simulink model "gm_sampleModel1847_2_sub_sub_sub"  (R2023a)
settings: Solver=VariableStepAuto  StartTime=0.0  StopTime=10.0  RelTol=1e-3
libraries: hdlsllib x3
settings Model: Creator=user1  LastModifiedBy=user1
settings OptimizationCC: BlockReduction=off  ConditionallyExecuteInputs=off
settings DebuggingCC: InheritedTsInSrcMsg=none

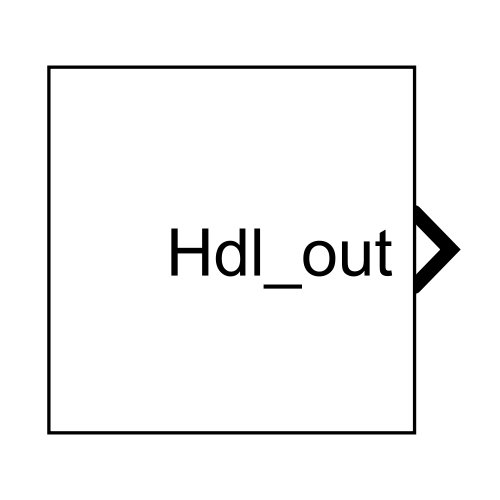
[thumbnail: Simulink's stored preview of the top-level diagram]
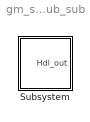
== system gm_sampleModel1847_2_sub_sub_sub ==
  Subsystem : Subsystem

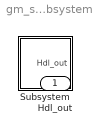
== system gm_sampleModel1847_2_sub_sub_sub/Subsystem ==
  Subsystem : Subsystem
  Hdl_out : Outport  OutDataTypeStr=uint8

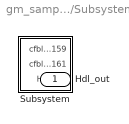
== system gm_sampleModel1847_2_sub_sub_sub/Subsystem/Subsystem ==
  Subsystem : Subsystem
  Hdl_out : Outport  OutDataTypeStr=uint8

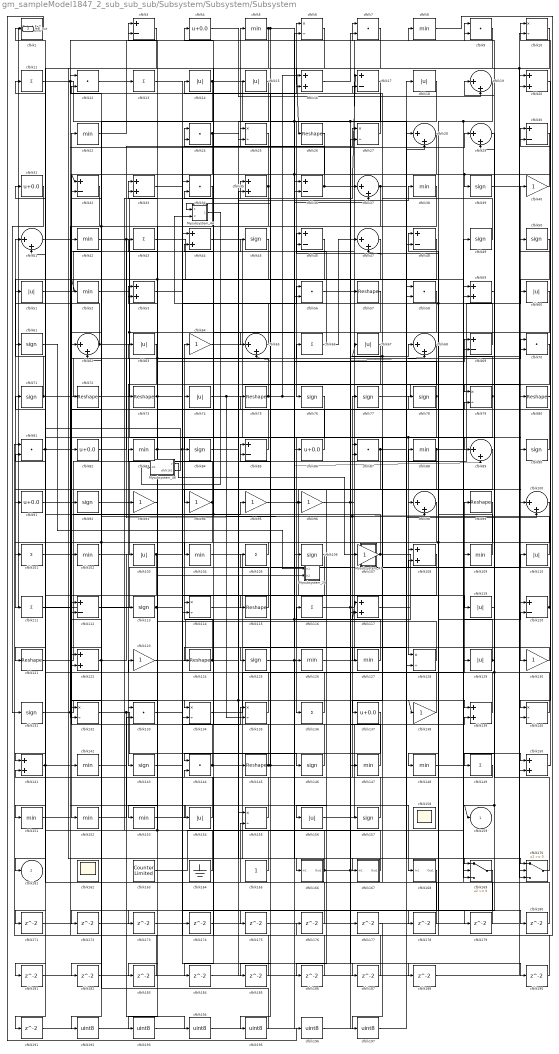
== system gm_sampleModel1847_2_sub_sub_sub/Subsystem/Subsystem/Subsystem ==
  Mysubsystem_26 : Subsystem  TreatAsAtomicUnit=on  RTWFcnName=Mysubsystem_26
      settings: RTWFcnNameOpts=User specified  RTWFileNameOpts=Use function name
  Mysubsystem_43 : Subsystem  TreatAsAtomicUnit=on  RTWFcnName=Mysubsystem_43
      settings: RTWFcnNameOpts=User specified  RTWFileNameOpts=Use function name
  Mysubsystem_44 : Subsystem  TreatAsAtomicUnit=on  RTWFcnName=Mysubsystem_44
      settings: RTWFcnNameOpts=User specified  RTWFileNameOpts=Use function name
  Mysubsystem_46 : Subsystem  TreatAsAtomicUnit=on  RTWFcnName=Mysubsystem_46
      settings: RTWFcnNameOpts=User specified  RTWFileNameOpts=Use function name
  cfblk1 : hdlsllib/Logic and Bit Operations/Detect Fall Nonpositive  vinit=0  OutDataTypeStr=uint8
  cfblk{6,10,25,27,79,114,128,132,134..135,140,155} (12 alike) : Product  Inputs=*/  OutDataTypeStr=uint8  RndMeth=Zero  SaturateOnIntegerOverflow=on
  cfblk{19,28..29,37,41,47,62,65,68,89,98,100} (12 alike) : Sum  Inputs=|++  OutDataTypeStr=uint8
  cfblk{11,13,43,66,101,105,111,116,136,149} (10 alike) : Sum  Inputs=+  OutDataTypeStr=uint8
  cfblk{5,8,22,38,42,52,83,88,102,104,109,126..127,142,147..148,151..153} (19 alike) : MinMax  OutDataTypeStr=uint8
  cfblk{14..15,18,51,60,63,67,74,103,110,119,129,154,156} (14 alike) : Abs  OutDataTypeStr=uint8  SaturateOnIntegerOverflow=off
  cfblk{39,45,49..50,61,71,76..78,84,90,92,106,113,125,131,143,146,157} (19 alike) : Signum
  cfblk{40,64,93..96,107,123,130,138} (10 alike) : Gain  OutDataTypeStr=uint8
  cfblk{16,20,33,35,44,53,59,108,117,122,139,141,150} (13 alike) : Sum  OutDataTypeStr=uint8
  cfblk{3,17,30,32,36,46,48,69,85,112,120} (11 alike) : Sum  Inputs=+-  OutDataTypeStr=uint8
  cfblk{26,57,72..73,75,80,99,115,121,124,145} (11 alike) : Reshape
  cfblk{7,9,12,24,34,56,58,70,81,87,133,144} (12 alike) : DotProduct  OutDataTypeStr=uint8
  cfblk{4,31,82,86,91,137} (6 alike) : Bias  Bias=0.0  SaturateOnIntegerOverflow=off
  cfblk158 : Scope
      settings: Floating=on
  cfblk162 : Scope
      settings: Floating=on
  cfblk163 : hdlsllib/Sources/Counter Limited  uplimit=7  tsamp=-1
  cfblk164 : Ground
  cfblk165 : Constant  OutDataTypeStr=uint8  SampleTime=-1
  cfblk166 : Subsystem
      settings: LibrarySourceBlock=|
      | hdlsllib/Ports &
      | Subsystems/Subsystem
  cfblk167 : Subsystem
      settings: LibrarySourceBlock=|
      | hdlsllib/Ports &
      | Subsystems/Subsystem
  cfblk168 : Subsystem
      settings: LibrarySourceBlock=|
      | hdlsllib/Ports &
      | Subsystems/Subsystem
  cfblk169 : Switch  OutDataTypeStr=uint8  SaturateOnIntegerOverflow=off  InputSameDT=off
  cfblk170 : Switch  OutDataTypeStr=uint8  SaturateOnIntegerOverflow=off  InputSameDT=off
  cfblk{171..188,190..191} (20 alike) : Delay  SampleTime=1
  cfblk{192..197} (6 alike) : DataTypeConversion  OutDataTypeStr=uint8  SaturateOnIntegerOverflow=off  RndMeth=Floor
  cfblk159 : Outport  OutDataTypeStr=uint8  VectorParamsAs1DForOutWhenUnconnected=off
  cfblk161 : Outport  Port=2  OutDataTypeStr=uint8  VectorParamsAs1DForOutWhenUnconnected=off
  Hdl_out : Outport  Port=3  OutDataTypeStr=uint8
  wires:
  Mysubsystem_46/2(cfblk161) -> cfblk161/1
  Mysubsystem_46/1(y) -> Mysubsystem_43/1(In1)
  Mysubsystem_44/1(Out1) -> Mysubsystem_46/1(In1)
  cfblk61/1 -> Mysubsystem_26/1(In1)
  cfblk197/1 -> cfblk58/2
  cfblk177/1 -> cfblk197/1
  cfblk196/1 -> cfblk58/1
  cfblk1/1 -> cfblk196/1
  cfblk195/1 -> cfblk42/1
  cfblk58/1 -> cfblk195/1
  cfblk194/1 -> cfblk28/2
  cfblk193/1 -> cfblk28/1
  cfblk192/1 -> cfblk177/1
  cfblk28/1 -> cfblk192/1
  cfblk191/1 -> cfblk56/2
  cfblk190/1 -> cfblk108/2
  cfblk188/1 -> cfblk120/1
  cfblk187/1 -> cfblk44/1
  cfblk33/1 -> cfblk187/1
  cfblk186/1 -> cfblk144/2
  cfblk98/1 -> cfblk186/1
  cfblk185/1 -> cfblk12/1
  cfblk169/1 -> cfblk185/1
  cfblk184/1 -> cfblk35/2
  cfblk9/1 -> cfblk184/1
  cfblk183/1 -> cfblk81/1
  cfblk182/1 -> cfblk10/2
  cfblk181/1 -> cfblk27/2
  cfblk180/1 -> cfblk59/1
  cfblk179/1 -> cfblk17/2
  cfblk178/1 -> cfblk1/1
  cfblk176/1 -> cfblk155/2
  cfblk8/1 -> cfblk176/1
  cfblk175/1 -> cfblk6/2
  cfblk57/1 -> cfblk175/1
  cfblk174/1 -> cfblk20/2
  cfblk133/1 -> cfblk174/1
  cfblk173/1 -> cfblk34/1
  cfblk93/1 -> cfblk173/1
  cfblk172/1 -> cfblk36/1
  cfblk168/1(Out1) -> cfblk172/1
  cfblk171/1 -> cfblk140/2
  cfblk84/1 -> cfblk167/1(In1), cfblk138/1
  cfblk130/1 -> cfblk124/1
  cfblk69/1 -> cfblk44/2
  cfblk63/1 -> cfblk73/1
  cfblk116/1 -> cfblk30/2, cfblk68/2
  cfblk142/1 -> cfblk169/1
  cfblk13/1 -> cfblk59/2
  cfblk127/1 -> cfblk116/1
  cfblk135/1 -> cfblk51/1
  cfblk4/1 -> cfblk19/2
  cfblk53/1 -> cfblk45/1
  cfblk67/1 -> cfblk115/1
  cfblk49/1 -> cfblk14/1
  cfblk150/1 -> cfblk30/1
  cfblk107/1 -> cfblk81/2, cfblk4/1, cfblk110/1
  cfblk14/1 -> cfblk48/2, cfblk147/1, cfblk132/1
  cfblk136/1 -> cfblk112/2
  cfblk51/1 -> cfblk18/1
  cfblk17/1 -> cfblk65/1
  cfblk83/1 -> cfblk27/1, cfblk96/1, cfblk3/2
  cfblk45/1 -> cfblk52/1, cfblk183/1
  cfblk110/1 -> cfblk87/2, cfblk62/2
  cfblk94/1 -> cfblk122/1, cfblk122/2, cfblk53/2
  cfblk15/1 -> cfblk25/2
  cfblk81/1 -> cfblk79/2, cfblk171/1
  cfblk19/1 -> cfblk148/1, cfblk169/2
  cfblk59/1 -> cfblk19/1
  cfblk111/1 -> cfblk69/1
  cfblk77/1 -> cfblk79/1
  cfblk26/1 -> cfblk36/2, cfblk62/1
  cfblk16/1 -> cfblk7/2
  cfblk75/1 -> cfblk128/2, cfblk16/1, Mysubsystem_26/2(In2), cfblk33/2
  cfblk22/1 -> cfblk7/1
  cfblk165/1 -> cfblk43/1, cfblk32/2
  cfblk65/1 -> cfblk34/2
  cfblk11/1 -> cfblk157/1, cfblk86/1, cfblk16/2
  cfblk41/1 -> cfblk29/1
  cfblk117/1 -> cfblk60/1
  cfblk47/1 -> cfblk134/2
  cfblk140/1 -> cfblk85/2, cfblk109/1
  cfblk70/1 -> cfblk125/1
  cfblk115/1 -> cfblk105/1
  cfblk48/1 -> cfblk102/1
  cfblk6/1 -> cfblk84/1
  cfblk109/1 -> Mysubsystem_44/2(In2), cfblk48/1
  cfblk163/1 -> cfblk129/1
  cfblk12/1 -> cfblk13/1
  cfblk156/1 -> cfblk49/1
  cfblk24/1 -> cfblk112/1, cfblk89/1
  cfblk104/1 -> cfblk127/1
  cfblk88/1 -> cfblk156/1, cfblk150/1
  cfblk90/1 -> cfblk33/1
  cfblk39/1 -> cfblk170/3
  cfblk108/1 -> cfblk151/1
  cfblk151/1 -> cfblk154/1
  cfblk128/1 -> cfblk3/1
  cfblk71/1 -> cfblk41/1, cfblk66/1
  cfblk34/1 -> cfblk113/1
  cfblk101/1 -> cfblk95/1
  cfblk66/1 -> cfblk46/1, cfblk47/1
  cfblk129/1 -> cfblk88/1, cfblk29/2
  cfblk31/1 -> cfblk131/1
  cfblk105/1 -> cfblk101/1
  cfblk95/1 -> cfblk119/1, cfblk100/1
  cfblk91/1 -> cfblk63/1
  cfblk37/1 -> cfblk93/1, cfblk100/2
  cfblk40/1 -> cfblk39/1, cfblk32/1
  cfblk120/1 -> cfblk50/1, cfblk75/1
  cfblk144/1 -> cfblk38/1, cfblk12/2
  cfblk113/1 -> cfblk56/1, Hdl_out/1
  cfblk7/1 -> cfblk91/1
  cfblk96/1 -> cfblk40/1, cfblk68/1, cfblk190/1
  cfblk92/1 -> cfblk70/2
  cfblk103/1 -> cfblk180/1, cfblk181/1
  cfblk25/1 -> cfblk24/2
  cfblk164/1 -> cfblk71/1
  cfblk148/1 -> cfblk120/2
  cfblk143/1 -> cfblk135/1
  cfblk72/1 -> cfblk70/1
  cfblk141/1 -> cfblk8/1, cfblk31/1
  cfblk5/1 -> Mysubsystem_44/1(In1), cfblk37/2, cfblk41/2
  cfblk52/1 -> cfblk114/2, cfblk106/1
  cfblk112/1 -> cfblk57/1
  cfblk123/1 -> cfblk20/1
  cfblk147/1 -> cfblk114/1
  cfblk29/1 -> cfblk149/1
  cfblk43/1 -> cfblk145/1
  cfblk86/1 -> cfblk25/1
  cfblk152/1 -> cfblk133/2
  cfblk89/1 -> cfblk98/1
  cfblk139/1 -> cfblk67/1, cfblk47/2
  cfblk79/1 -> cfblk137/1, cfblk46/2
  cfblk149/1 -> cfblk141/2
  cfblk74/1 -> cfblk108/1, cfblk135/2
  cfblk166/1(Out1) -> cfblk139/2, cfblk188/1, cfblk61/1
  cfblk60/1 -> cfblk94/1
  cfblk138/1 -> cfblk92/1
  cfblk121/1 -> cfblk87/1
  cfblk100/1 -> cfblk104/1
  cfblk122/1 -> cfblk103/1, cfblk182/1
  cfblk20/1 -> cfblk140/1
  cfblk62/1 -> cfblk37/1, cfblk11/1
  cfblk125/1 -> cfblk170/2, cfblk69/2
  cfblk106/1 -> cfblk121/1
  cfblk10/1 -> cfblk26/1, cfblk150/2
  cfblk137/1 -> cfblk144/1
  cfblk38/1 -> cfblk153/1
  cfblk82/1 -> cfblk24/1
  cfblk80/1 -> cfblk10/1
  cfblk42/1 -> cfblk155/1, cfblk98/2
  cfblk145/1 -> cfblk89/2, cfblk117/1, cfblk126/1, cfblk65/2, cfblk72/1
  cfblk56/1 -> cfblk107/1
  cfblk154/1 -> cfblk83/1
  cfblk119/1 -> cfblk159/1, cfblk179/1
  cfblk44/1 -> cfblk90/1
  cfblk32/1 -> cfblk142/1
  cfblk114/1 -> cfblk170/1
  cfblk73/1 -> cfblk133/1, cfblk117/2
  cfblk102/1 -> cfblk85/1
  cfblk76/1 -> cfblk136/1
  cfblk155/1 -> cfblk123/1
  cfblk146/1 -> cfblk22/1
  cfblk157/1 -> cfblk77/1
  cfblk124/1 -> cfblk74/1, cfblk78/1
  cfblk27/1 -> cfblk6/1
  cfblk170/1 -> cfblk9/2
  cfblk87/1 -> cfblk141/1, cfblk169/3
  cfblk36/1 -> cfblk17/1, cfblk15/1
  cfblk126/1 -> cfblk9/1
  cfblk35/1 -> cfblk132/2, cfblk82/1, cfblk5/1
  cfblk131/1 -> cfblk134/1, cfblk139/1
  cfblk18/1 -> cfblk76/1
  cfblk153/1 -> cfblk168/1(In1)
  cfblk46/1 -> cfblk111/1
  cfblk99/1 -> cfblk178/1, cfblk193/1
  cfblk132/1 -> cfblk146/1, cfblk194/1
  cfblk167/1(Out1) -> cfblk35/1
  cfblk3/1 -> cfblk166/1(In1)
  cfblk30/1 -> cfblk152/1
  cfblk134/1 -> cfblk99/1
  cfblk78/1 -> cfblk128/1, cfblk191/1, cfblk53/1
  cfblk85/1 -> cfblk64/1
  cfblk64/1 -> cfblk80/1
  cfblk68/1 -> cfblk143/1
  cfblk50/1 -> cfblk130/1

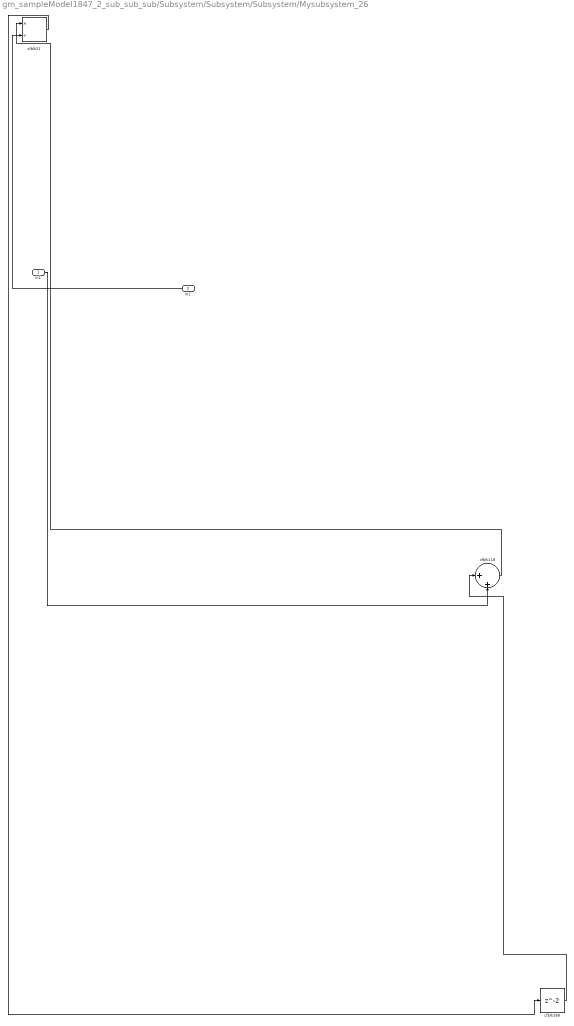
== system gm_sampleModel1847_2_sub_sub_sub/Subsystem/Subsystem/Subsystem/Mysubsystem_26 ==
  In1 : Inport
  In2 : Inport  Port=2
  cfblk118 : Sum  Inputs=|++
  cfblk189 : Delay  SampleTime=1
  cfblk21 : Product  Inputs=*/  RndMeth=Zero  SaturateOnIntegerOverflow=on
  wires:
  cfblk118/1 -> cfblk21/1
  cfblk21/1 -> cfblk189/1
  cfblk189/1 -> cfblk118/1
  In1/1 -> cfblk118/2
  In2/1 -> cfblk21/2

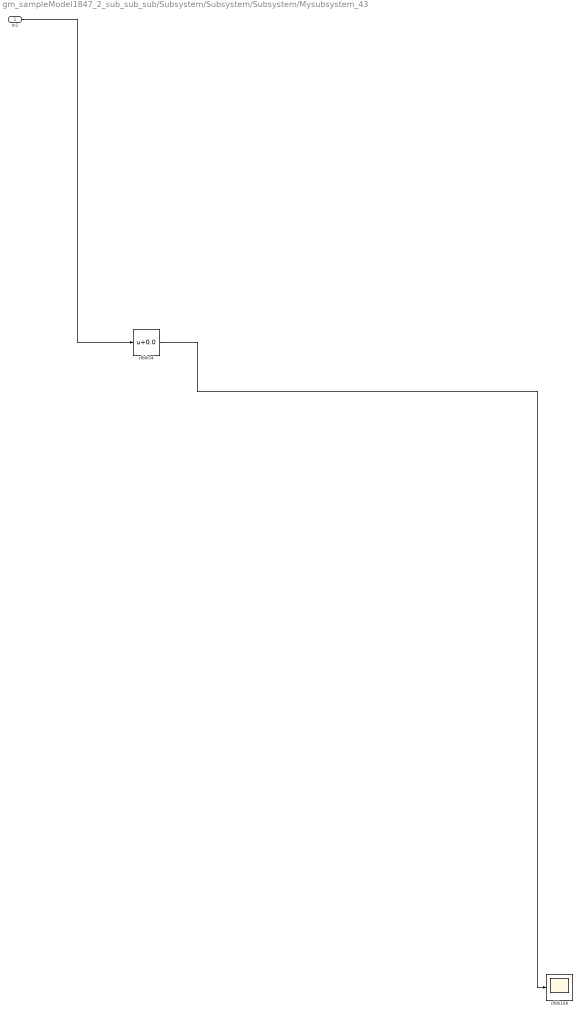
== system gm_sampleModel1847_2_sub_sub_sub/Subsystem/Subsystem/Subsystem/Mysubsystem_43 ==
  In1 : Inport
  cfblk160 : Scope
  cfblk54 : Bias  Bias=0.0  SaturateOnIntegerOverflow=off
  wires:
  cfblk54/1 -> cfblk160/1
  In1/1 -> cfblk54/1

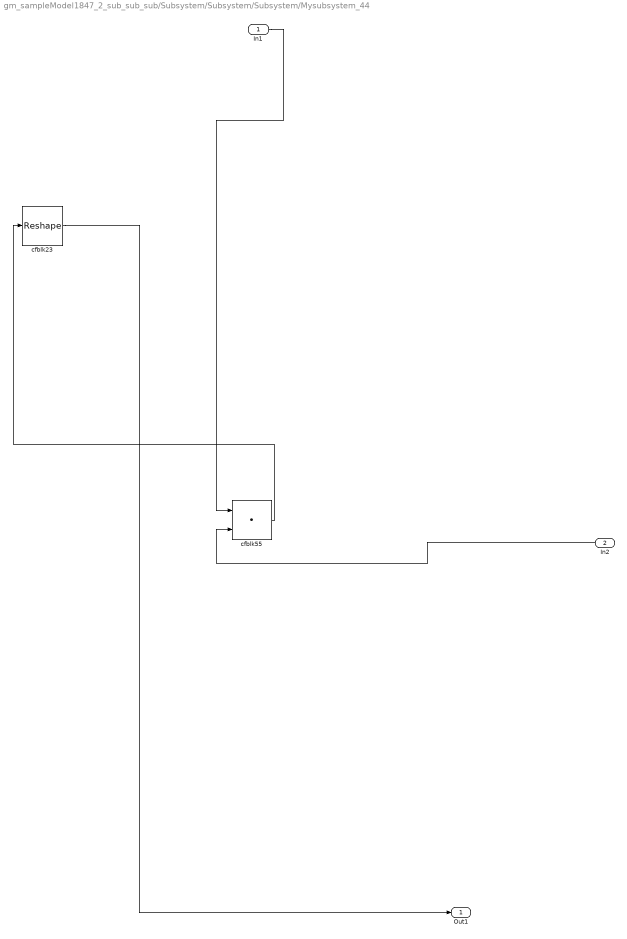
== system gm_sampleModel1847_2_sub_sub_sub/Subsystem/Subsystem/Subsystem/Mysubsystem_44 ==
  In1 : Inport
  In2 : Inport  Port=2
  cfblk23 : Reshape
  cfblk55 : DotProduct  OutDataTypeStr=Inherit: Inherit via internal rule
  Out1 : Outport
  wires:
  cfblk55/1 -> cfblk23/1
  cfblk23/1 -> Out1/1
  In2/1 -> cfblk55/2
  In1/1 -> cfblk55/1

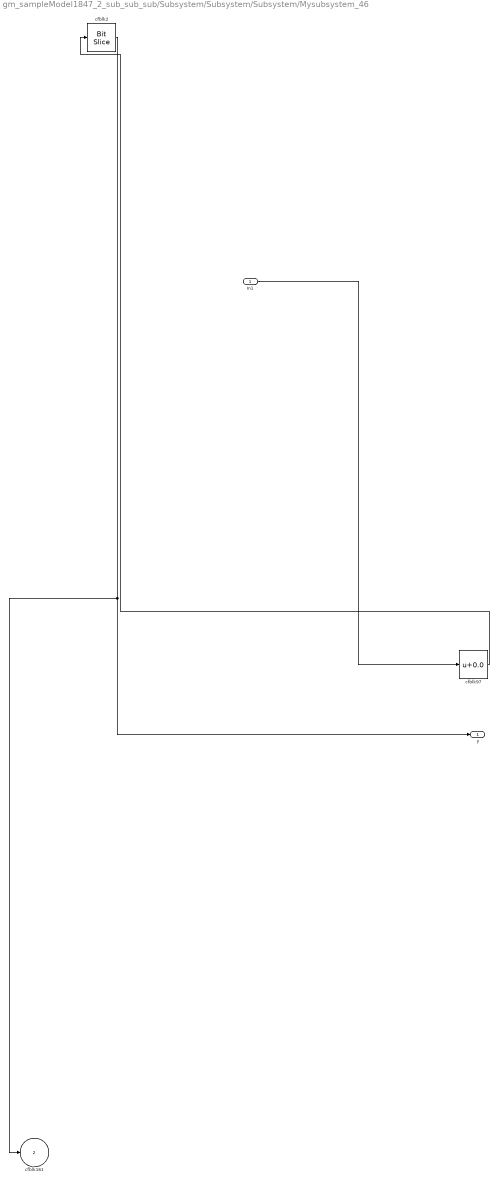
== system gm_sampleModel1847_2_sub_sub_sub/Subsystem/Subsystem/Subsystem/Mysubsystem_46 ==
  In1 : Inport
  cfblk2 : hdlsllib/Logic and Bit Operations/Bit Slice  lidx=7  ridx=0
  cfblk97 : Bias  Bias=0.0  SaturateOnIntegerOverflow=off
  y : Outport
  cfblk161 : Outport  Port=2  VectorParamsAs1DForOutWhenUnconnected=off
  wires:
  cfblk97/1 -> cfblk2/1
  cfblk2/1 -> cfblk161/1, y/1
  In1/1 -> cfblk97/1

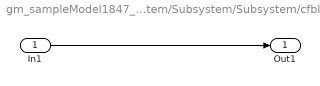
== system gm_sampleModel1847_2_sub_sub_sub/Subsystem/Subsystem/Subsystem/cfblk166 ==
  In1 : Inport
  Out1 : Outport
  wires:
  In1/1 -> Out1/1

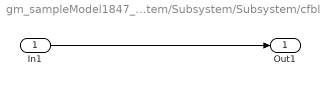
== system gm_sampleModel1847_2_sub_sub_sub/Subsystem/Subsystem/Subsystem/cfblk167 ==
  In1 : Inport
  Out1 : Outport
  wires:
  In1/1 -> Out1/1

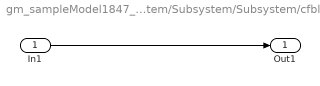
== system gm_sampleModel1847_2_sub_sub_sub/Subsystem/Subsystem/Subsystem/cfblk168 ==
  In1 : Inport
  Out1 : Outport
  wires:
  In1/1 -> Out1/1
